simulink model "Q4_Two_Mass"  (R2026a)
settings: Solver=ode45  StopTime=12  RelTol=1e-8  AbsTol=1e-10
settings Model: Creator=szj  LastModifiedBy=szj

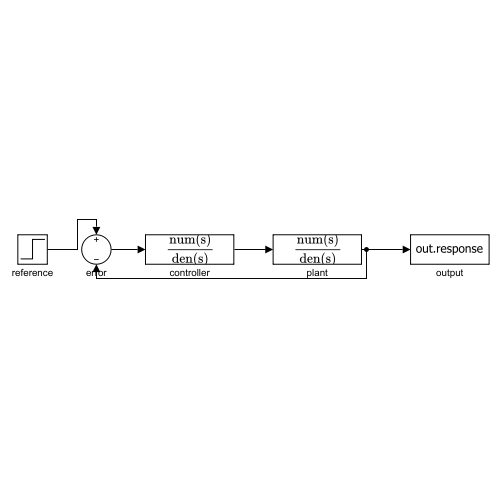
[thumbnail: Simulink's stored preview of the top-level diagram]
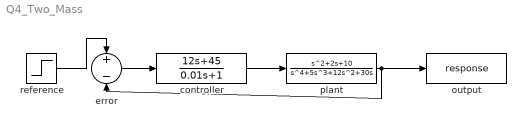
== system Q4_Two_Mass ==
  controller : TransferFcn  Numerator=[12 45]  Denominator=[0.01 1]
  error : Sum  Inputs=+-
  output : ToWorkspace  VariableName=response  SaveFormat=Timeseries  SampleTime=-1
  plant : TransferFcn  Numerator=[0 0 1 2 10]  Denominator=[1 5 12 30 0]
  reference : Step  SampleTime=0
  wires:
  reference/1 -> error/1
  error/1 -> controller/1
  controller/1 -> plant/1
  plant/1 -> output/1, error/2
